simulink model "bh_2dof_NP_CONTROLLED_compare_lagr_sm"  (R2017a)
settings: Solver=ode45  StartTime=0.0  StopTime=70  FixedStep=0.001  RelTol=1e-7  EnableMultiTasking=on
values from neighbouring files (symbols this model uses):
  theta1_0 = 0    [bh_SIMPARAMS_for_2dof_NP_Control_sim.m]
  theta1_dot_0 = 0    [bh_SIMPARAMS_for_2dof_NP_Control_sim.m]
  theta4_0 = 0    [bh_SIMPARAMS_for_2dof_NP_Control_sim.m]
  theta4_dot_0 = 0    [bh_SIMPARAMS_for_2dof_NP_Control_sim.m]
undefined symbols (not defined in the file or in its folder): b1_damp, b4_damp, g, Hz, L1x, L1y, L1z, mass1, mass4, Rturn, sigbuilder_block, X, Y, Z
libraries: simulink_extras x30, sm_lib x13, nesl_utility x9, simulink x8, discretizing x2
(part 1 of 2)
settings Model: Creator=bhorton  LastModifiedBy=bhorton
settings SolverCC: ZeroCrossAlgorithm=Adaptive
settings OptimizationCC: LifeSpan=inf
settings DebuggingCC: SFUnexpectedBacktrackingDiag=warning  SFNoUnconditionalDefaultTransitionDiag=warning  SFExecutionAtInitializationDiag=none
settings GRTTargetCC: TargetLangStandard=C89/C90 (ANSI)
settings ConfigComp: CovMetricSettings=dw  CovHtmlReporting=on  CovSaveCumulativeToWorkspaceVar=on  CovSaveSingleToWorkspaceVar=on  CovExternalEMLEnable=off
settings SimscapeCC: SimscapeLogDataHistory=10000  SelectedTab=Simscape Multibody
settings ExplorerConfigSet: InternalSimMechanicsExplorerSettings="<ExplorerConfiguration><canonicalview>default</canonicalview><AnimationSetting><BasePlaybackSpeed>2</BasePlaybackSpeed><PlaybackSpeedFactor>1.0</PlaybackSpeedFactor></AnimationSetting><TilePanel><TileInfo><Tiles Columns=\"1\" Count=\"1\" Rows=\"1\"><Column Left=\"2\" Weight=\"1\"/><Column Left=\"820\"/><Row Top=\"2\" Weight=\"1\"/><Row Top=\"545\"/><Tile Height=\"1\" Width=\"1\" X=\"0\" Y=\"0\"/></Tiles></TileInfo><SceneInfo><SceneViewer><BGColor><R>0.60000002384185791</R><G>0.60000002384185791</G><B>0.60000002384185791</B></BGColor><Camera><DoPerspective>off</DoPerspective><Position><X>0.3018347345439823</X><Y>0.024415264242792611</Y><Z>0.21433472519445274</Z></Position><Center><X>0.024999999062628675</X><Y>0.30124999972414623</Y><Z>-0.062500010286905439</Z></Center><Up><X>-0.40824829046386751</X><Y>0.40824829046386751</Y><Z>0.81649658092772159</Z></Up><ViewLimDist>1</ViewLimDist><YLim>0.27384785473346712</YLim><XLim>0.4148743716842227</XLim></Camera></SceneViewer></SceneInfo></TilePanel><MechEditorPanel><Cameras/><GfxPanelCameraMap/></MechEditorPanel></ExplorerConfiguration>"

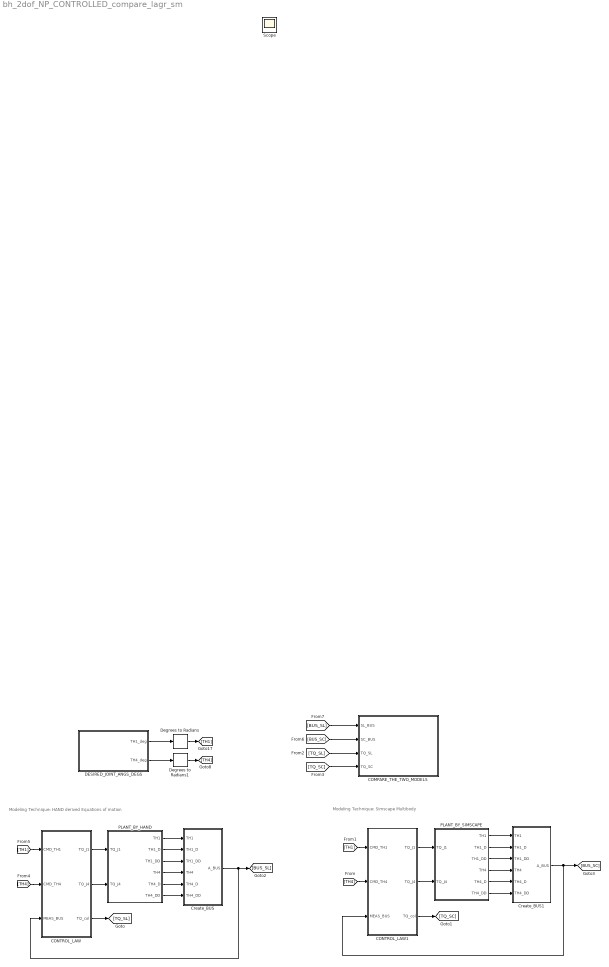
== system bh_2dof_NP_CONTROLLED_compare_lagr_sm ==
  note: Modeling Technique: Simscape Multibody
  note: Modeling Technique: HAND derived Equations of motion
  COMPARE_THE_TWO_MODELS : Subsystem
  CONTROL_LAW : Subsystem
  CONTROL_LAW1 : Subsystem
  Create_BUS : Subsystem
  Create_BUS1 : Subsystem
  DESIRED_JOINT_ANGS_DEGS : Subsystem  Tag=STV Subsys  LoadFcn=sigbuilder_block('load');  StartFcn=sigbuilder_block('start');  StopFcn=sigbuilder_block('stop');  ClipboardFcn=sigbuilder_block('clipboard');  mask(Sigbuilder block){tuvar=[0:10]}
      mask help: Simulink:masks:SigbuilderBlock_MD
      mask init:
      | if ~strcmp(get_param(bdroot(gcbh),'SimulationStatus'),'stopped') tuvar = sigbuilder_block('maskInit'); end
      settings: CopyFcn=sigbuilder_block('copy');  DeleteFcn=sigbuilder_block('delete');  ModelCloseFcn=sigbuilder_block('modelClose');  PreSaveFcn=sigbuilder_block('preSave');  PauseFcn=sigbuilder_block('pause');  ContinueFcn=sigbuilder_block('continue');  NameChangeFcn=sigbuilder_block('namechange');  OpenFcn=sigbuilder_block('open',[6 30 1428 681.75 ]);  CloseFcn=sigbuilder_block('close');
      mask Display: plot(0, 0, 100, 100,[2, 2, 32, 32, 2], [68, 8, 8, 68, 68],[32, 2], [38, 38], [32, 19, 2],[53, 60, 44], [32, 17, 17, 2],[16, 16, 31, 31]);txt = getActiveGroup(gcbh);text(2, 100, txt,'verticalAlignment', 'top');
  Degrees to Radians : simulink_extras/Transformations/Degrees to Radians
  Degrees to Radians1 : simulink_extras/Transformations/Degrees to Radians
  PLANT_BY_HAND : Subsystem
  PLANT_BY_SIMSCAPE : Subsystem
  Scope : Scope
  wires:
  DESIRED_JOINT_ANGS_DEGS/2(TH4_deg) -> Degrees to Radians1/1
  DESIRED_JOINT_ANGS_DEGS/1(TH1_deg) -> Degrees to Radians/1
  Degrees to Radians/1 -> [TH1]
  Degrees to Radians1/1 -> [TH4]
  CONTROL_LAW/1(TQ_J1) -> PLANT_BY_HAND/1("TQ_J1 ")
  Create_BUS/1(A_BUS) -> [BUS_SL], CONTROL_LAW/3(MEAS_BUS)
  PLANT_BY_HAND/4(TH4) -> Create_BUS/4(TH4)
  PLANT_BY_HAND/6(TH4_DD) -> Create_BUS/6(TH4_DD)
  PLANT_BY_HAND/1(TH1) -> Create_BUS/1(TH1)
  PLANT_BY_HAND/2(TH1_D) -> Create_BUS/2(TH1_D)
  PLANT_BY_HAND/3(TH1_DD) -> Create_BUS/3(TH1_DD)
  PLANT_BY_HAND/5(TH4_D) -> Create_BUS/5(TH4_D)
  PLANT_BY_SIMSCAPE/1(TH1) -> Create_BUS1/1(TH1)
  PLANT_BY_SIMSCAPE/2(TH1_D) -> Create_BUS1/2(TH1_D)
  PLANT_BY_SIMSCAPE/3(TH1_DD) -> Create_BUS1/3(TH1_DD)
  PLANT_BY_SIMSCAPE/4(TH4) -> Create_BUS1/4(TH4)
  PLANT_BY_SIMSCAPE/5(TH4_D) -> Create_BUS1/5(TH4_D)
  PLANT_BY_SIMSCAPE/6(TH4_DD) -> Create_BUS1/6(TH4_DD)
  Create_BUS1/1(A_BUS) -> [BUS_SC], CONTROL_LAW1/3(MEAS_BUS)
  CONTROL_LAW1/1(TQ_J1) -> PLANT_BY_SIMSCAPE/1("TQ_J1 ")
  CONTROL_LAW1/2(TQ_J4) -> PLANT_BY_SIMSCAPE/2(TQ_J4)
  [TH4] -> CONTROL_LAW1/2(CMD_TH4)
  [TH1] -> CONTROL_LAW1/1(CMD_TH1)
  CONTROL_LAW/3(TQ_col) -> [TQ_SL]
  CONTROL_LAW1/3(TQ_col) -> [TQ_SC]
  [TQ_SC] -> COMPARE_THE_TWO_MODELS/4(TQ_SC)
  [TQ_SL] -> COMPARE_THE_TWO_MODELS/3(TQ_SL)
  [TH4] -> CONTROL_LAW/2(CMD_TH4)
  [TH1] -> CONTROL_LAW/1(CMD_TH1)
  [BUS_SC] -> COMPARE_THE_TWO_MODELS/2(SC_BUS)
  [BUS_SL] -> COMPARE_THE_TWO_MODELS/1(SL_BUS)
  CONTROL_LAW/2(TQ_J4) -> PLANT_BY_HAND/2(TQ_J4)

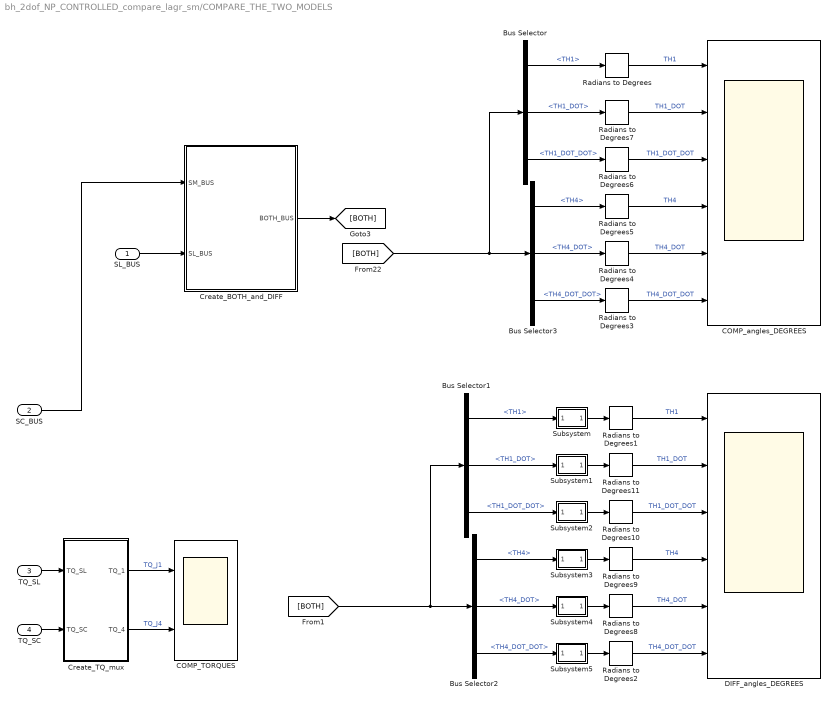
== system bh_2dof_NP_CONTROLLED_compare_lagr_sm/COMPARE_THE_TWO_MODELS ==
  SL_BUS : Inport
  SC_BUS : Inport  Port=2
  TQ_SL : Inport  Port=3
  TQ_SC : Inport  Port=4
  Bus Selector : BusSelector  OutputSignals=TH1,TH1_DOT,TH1_DOT_DOT
  Bus Selector1 : BusSelector  OutputSignals=TH1,TH1_DOT,TH1_DOT_DOT
  Bus Selector2 : BusSelector  OutputSignals=TH4,TH4_DOT,TH4_DOT_DOT
  Bus Selector3 : BusSelector  OutputSignals=TH4,TH4_DOT,TH4_DOT_DOT
  COMP_TORQUES : Scope  NumInputPorts=2
  COMP_angles_DEGREES : Scope  NumInputPorts=6
  Create_BOTH_and_DIFF : Subsystem
  Create_TQ_mux : Subsystem
  DIFF_angles_DEGREES : Scope  NumInputPorts=6
  Radians to Degrees{,1..11} (12 alike) : simulink_extras/Transformations/Radians to Degrees
  Subsystem : Subsystem
  Subsystem1 : Subsystem
  Subsystem2 : Subsystem
  Subsystem3 : Subsystem
  Subsystem4 : Subsystem
  Subsystem5 : Subsystem
  wires:
  SC_BUS/1 -> Create_BOTH_and_DIFF/1(SM_BUS)
  SL_BUS/1 -> Create_BOTH_and_DIFF/2(SL_BUS)
  Create_BOTH_and_DIFF/1(BOTH_BUS) -> [BOTH]
  Bus Selector/1 -> Radians to Degrees/1  "<TH1>"
  Bus Selector/2 -> Radians to Degrees7/1  "<TH1_DOT>"
  Bus Selector/3 -> Radians to Degrees6/1  "<TH1_DOT_DOT>"
  Bus Selector3/1 -> Radians to Degrees5/1  "<TH4>"
  Bus Selector3/2 -> Radians to Degrees4/1  "<TH4_DOT>"
  Bus Selector3/3 -> Radians to Degrees3/1  "<TH4_DOT_DOT>"
  [BOTH] -> Bus Selector/1, Bus Selector3/1
  Radians to Degrees/1 -> COMP_angles_DEGREES/1  "TH1"
  Radians to Degrees7/1 -> COMP_angles_DEGREES/2  "TH1_DOT"
  Radians to Degrees6/1 -> COMP_angles_DEGREES/3  "TH1_DOT_DOT"
  Radians to Degrees5/1 -> COMP_angles_DEGREES/4  "TH4"
  Radians to Degrees4/1 -> COMP_angles_DEGREES/5  "TH4_DOT"
  Radians to Degrees3/1 -> COMP_angles_DEGREES/6  "TH4_DOT_DOT"
  Bus Selector1/1 -> Subsystem/1(In1)  "<TH1>"
  Bus Selector1/2 -> Subsystem1/1(In1)  "<TH1_DOT>"
  Bus Selector1/3 -> Subsystem2/1(In1)  "<TH1_DOT_DOT>"
  Bus Selector2/1 -> Subsystem3/1(In1)  "<TH4>"
  Bus Selector2/2 -> Subsystem4/1(In1)  "<TH4_DOT>"
  Bus Selector2/3 -> Subsystem5/1(In1)  "<TH4_DOT_DOT>"
  [BOTH] -> Bus Selector1/1, Bus Selector2/1
  Radians to Degrees1/1 -> DIFF_angles_DEGREES/1  "TH1"
  Radians to Degrees11/1 -> DIFF_angles_DEGREES/2  "TH1_DOT"
  Radians to Degrees10/1 -> DIFF_angles_DEGREES/3  "TH1_DOT_DOT"
  Radians to Degrees9/1 -> DIFF_angles_DEGREES/4  "TH4"
  Radians to Degrees8/1 -> DIFF_angles_DEGREES/5  "TH4_DOT"
  Radians to Degrees2/1 -> DIFF_angles_DEGREES/6  "TH4_DOT_DOT"
  Subsystem/1(diff) -> Radians to Degrees1/1
  Subsystem5/1(diff) -> Radians to Degrees2/1
  Subsystem4/1(diff) -> Radians to Degrees8/1
  Subsystem3/1(diff) -> Radians to Degrees9/1
  Subsystem2/1(diff) -> Radians to Degrees10/1
  Subsystem1/1(diff) -> Radians to Degrees11/1
  TQ_SC/1 -> Create_TQ_mux/2(TQ_SC)
  TQ_SL/1 -> Create_TQ_mux/1(TQ_SL)
  Create_TQ_mux/1(TQ_1) -> COMP_TORQUES/1  "TQ_J1"
  Create_TQ_mux/2(TQ_4) -> COMP_TORQUES/2  "TQ_J4"

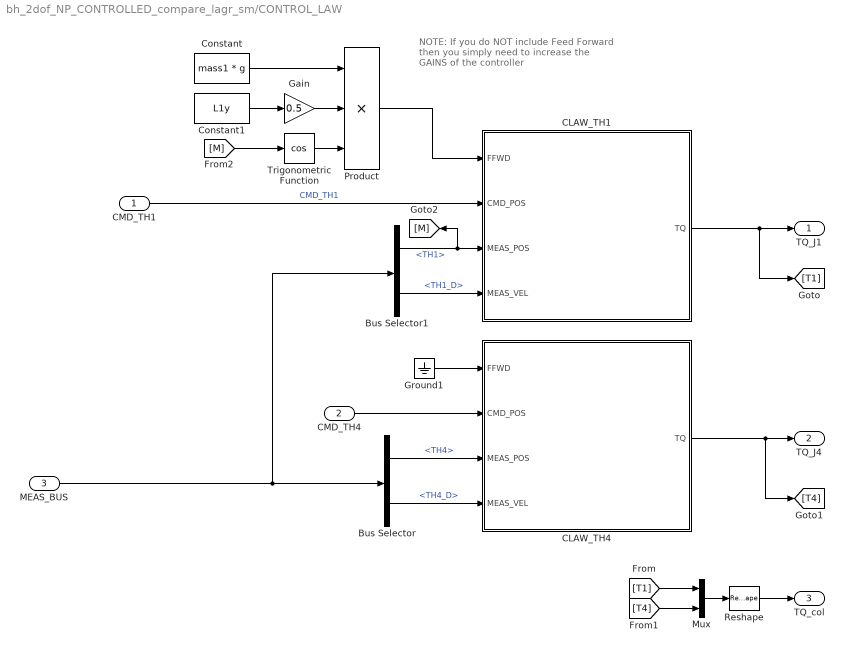
== system bh_2dof_NP_CONTROLLED_compare_lagr_sm/CONTROL_LAW ==
  note: NOTE:
      | If you do NOT include Feed Forward
      | then you simply need to increase the GAINS of the controller
  CMD_TH1 : Inport
  CMD_TH4 : Inport  Port=2
  MEAS_BUS : Inport  Port=3
  Bus Selector : BusSelector  OutputSignals=TH4,TH4_D
  Bus Selector1 : BusSelector  OutputSignals=TH1,TH1_D
  CLAW_TH1 : Subsystem
  CLAW_TH4 : Subsystem
  Constant : Constant  Value=mass1 * g
  Constant1 : Constant  Value=L1y
  Gain : Gain  Gain=0.5
  Ground1 : Ground
  Mux : Mux  Inputs=2
  Product : Product  Inputs=3
  Reshape : Reshape  OutputDimensionality=Column vector (2-D)
  Trigonometric Function : Trigonometry  Operator=cos
  TQ_J1 : Outport
  TQ_J4 : Outport  Port=2
  TQ_col : Outport  Port=3
  wires:
  MEAS_BUS/1 -> Bus Selector1/1, Bus Selector/1
  CMD_TH4/1 -> CLAW_TH4/2(CMD_POS)
  Bus Selector/2 -> CLAW_TH4/4(MEAS_VEL)  "<TH4_D>"
  Bus Selector/1 -> CLAW_TH4/3(MEAS_POS)  "<TH4>"
  Bus Selector1/1 -> [M], CLAW_TH1/3(MEAS_POS)  "<TH1>"
  Bus Selector1/2 -> CLAW_TH1/4(MEAS_VEL)  "<TH1_D>"
  CLAW_TH1/1(TQ) -> [T1], TQ_J1/1
  Ground1/1 -> CLAW_TH4/1(FFWD)
  CLAW_TH4/1(TQ) -> [T4], TQ_J4/1
  CMD_TH1/1 -> CLAW_TH1/2(CMD_POS)  "CMD_TH1"
  Constant/1 -> Product/1
  Constant1/1 -> Gain/1
  Product/1 -> CLAW_TH1/1(FFWD)
  Gain/1 -> Product/2
  Trigonometric Function/1 -> Product/3
  Mux/1 -> Reshape/1
  [T1] -> Mux/1
  [T4] -> Mux/2
  Reshape/1 -> TQ_col/1
  [M] -> Trigonometric Function/1

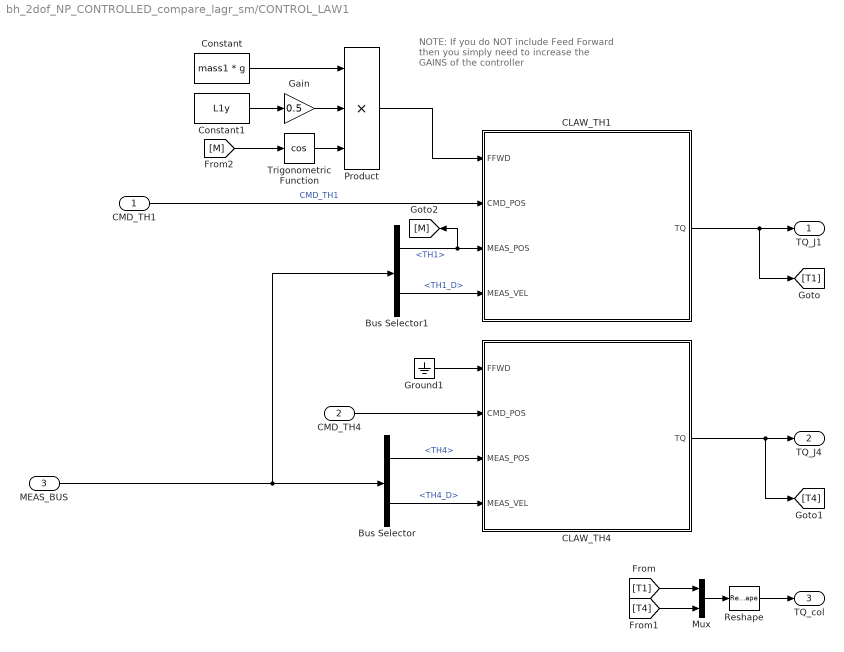
== system bh_2dof_NP_CONTROLLED_compare_lagr_sm/CONTROL_LAW1 ==
  note: NOTE:
      | If you do NOT include Feed Forward
      | then you simply need to increase the GAINS of the controller
  CMD_TH1 : Inport
  CMD_TH4 : Inport  Port=2
  MEAS_BUS : Inport  Port=3
  Bus Selector : BusSelector  OutputSignals=TH4,TH4_D
  Bus Selector1 : BusSelector  OutputSignals=TH1,TH1_D
  CLAW_TH1 : Subsystem
  CLAW_TH4 : Subsystem
  Constant : Constant  Value=mass1 * g
  Constant1 : Constant  Value=L1y
  Gain : Gain  Gain=0.5
  Ground1 : Ground
  Mux : Mux  Inputs=2
  Product : Product  Inputs=3
  Reshape : Reshape  OutputDimensionality=Column vector (2-D)
  Trigonometric Function : Trigonometry  Operator=cos
  TQ_J1 : Outport
  TQ_J4 : Outport  Port=2
  TQ_col : Outport  Port=3
  wires:
  MEAS_BUS/1 -> Bus Selector1/1, Bus Selector/1
  CMD_TH4/1 -> CLAW_TH4/2(CMD_POS)
  Bus Selector/2 -> CLAW_TH4/4(MEAS_VEL)  "<TH4_D>"
  Bus Selector/1 -> CLAW_TH4/3(MEAS_POS)  "<TH4>"
  Bus Selector1/1 -> [M], CLAW_TH1/3(MEAS_POS)  "<TH1>"
  Bus Selector1/2 -> CLAW_TH1/4(MEAS_VEL)  "<TH1_D>"
  CLAW_TH1/1(TQ) -> [T1], TQ_J1/1
  Ground1/1 -> CLAW_TH4/1(FFWD)
  CLAW_TH4/1(TQ) -> [T4], TQ_J4/1
  CMD_TH1/1 -> CLAW_TH1/2(CMD_POS)  "CMD_TH1"
  Constant/1 -> Product/1
  Constant1/1 -> Gain/1
  Product/1 -> CLAW_TH1/1(FFWD)
  Gain/1 -> Product/2
  Trigonometric Function/1 -> Product/3
  Mux/1 -> Reshape/1
  [T1] -> Mux/1
  [T4] -> Mux/2
  Reshape/1 -> TQ_col/1
  [M] -> Trigonometric Function/1

== system bh_2dof_NP_CONTROLLED_compare_lagr_sm/Create_BUS ==
  TH1 : Inport
  TH1_D : Inport  Port=2
  TH1_DD : Inport  Port=3
  TH4 : Inport  Port=4
  TH4_D : Inport  Port=5
  TH4_DD : Inport  Port=6
  Bus Creator : BusCreator  Inputs=6
  A_BUS : Outport
  wires:
  TH1_DD/1 -> Bus Creator/3  "TH1_DD"
  TH1_D/1 -> Bus Creator/2  "TH1_D"
  TH1/1 -> Bus Creator/1  "TH1"
  Bus Creator/1 -> A_BUS/1
  TH4_DD/1 -> Bus Creator/6  "TH4_DD"
  TH4_D/1 -> Bus Creator/5  "TH4_D"
  TH4/1 -> Bus Creator/4  "TH4"

== system bh_2dof_NP_CONTROLLED_compare_lagr_sm/Create_BUS1 ==
  TH1 : Inport
  TH1_D : Inport  Port=2
  TH1_DD : Inport  Port=3
  TH4 : Inport  Port=4
  TH4_D : Inport  Port=5
  TH4_DD : Inport  Port=6
  Bus Creator : BusCreator  Inputs=6
  A_BUS : Outport
  wires:
  TH1_DD/1 -> Bus Creator/3  "TH1_DD"
  TH1_D/1 -> Bus Creator/2  "TH1_D"
  TH1/1 -> Bus Creator/1  "TH1"
  Bus Creator/1 -> A_BUS/1
  TH4_DD/1 -> Bus Creator/6  "TH4_DD"
  TH4_D/1 -> Bus Creator/5  "TH4_D"
  TH4/1 -> Bus Creator/4  "TH4"

== system bh_2dof_NP_CONTROLLED_compare_lagr_sm/DESIRED_JOINT_ANGS_DEGS ==
  Demux : Demux  Tag=STV Demux  Outputs=2
  FromWs : FromWorkspace  Tag=STV FromWs  VariableName=tuvar  SampleTime=0
      SigBuilderData=|
      | common.afterFinalStr = 'Extrapolate'
      | common.sampleTime = 0
      | dataSet(1).timeRange = [0 60]
      | dataSet(1).name = 'SCENARIO_A_JUST_TH1'
      | dataSet(2).timeRange = [0 60]
      | dataSet(2).name = 'SCENARIO_B_JUST_TH4'
      | dataSet(3).timeRange = [0 60]
      | dataSet(3).name = 'SCENARIO_C_TH1_and_TH4'
      | dataSet(4).timeRange = [0 60]
      | dataSet(4).name = 'SCENARIO_D_TH1_and_TH4'
      | dataSet(5).timeRange = [0 70]
      | dataSet(5).name = 'SCENARIO_E'
      | sbobj.Groups(1).Name = 'SCENARIO_A_JUST_TH1'
      | sbobj.Groups(1).Signals(1).Name = 'TH1_deg'
      | sbobj.Groups(1).Signals(1).XData = [0 20 20 60]
      | sbobj.Groups(1).Signals(1).YData = [0 0 45 45]
      | sbobj.Groups(1).Signals(2).Name = 'TH4_deg'
      | sbobj.Groups(1).Signals(2).XData = [0 60]
      | sbobj.Groups(1).Signals(2).YData = [0 0]
      | sbobj.Groups(1).TimeRange = [0 60]
      | sbobj.Groups(2).Name = 'SCENARIO_B_JUST_TH4'
      | sbobj.Groups(2).Signals(1).Name = 'TH1_deg'
      | sbobj.Groups(2).Signals(1).XData = [0 20 60]
      | sbobj.Groups(2).Signals(1).YData = [0 0 0]
      | sbobj.Groups(2).Signals(2).Name = 'TH4_deg'
      | sbobj.Groups(2).Signals(2).XData = [0 20 20 60]
      | sbobj.Groups(2).Signals(2).YData = [0 0 45 45]
      | sbobj.Groups(2).TimeRange = [0 60]
      | sbobj.Groups(3).Name = 'SCENARIO_C_TH1_and_TH4'
      | sbobj.Groups(3).Signals(1).Name = 'TH1_deg'
      | sbobj.Groups(3).Signals(1).XData = [0 10 10 40 60]
      | sbobj.Groups(3).Signals(1).YData = [0 0 45 45 0]
      | sbobj.Groups(3).Signals(2).Name = 'TH4_deg'
      | sbobj.Groups(3).Signals(2).XData = [0 14.95 14.95 30 60]
      | sbobj.Groups(3).Signals(2).YData = [0 0 45 45 0]
      | sbobj.Groups(3).TimeRange = [0 60]
      | sbobj.Groups(4).Name = 'SCENARIO_D_TH1_and_TH4'
      | sbobj.Groups(4).Signals(1).Name = 'TH1_deg'
      | sbobj.Groups(4).Signals(1).XData = [0 10 40 60]
      | sbobj.Groups(4).Signals(1).YData = [0 45 45 0]
      | sbobj.Groups(4).Signals(2).Name = 'TH4_deg'
      | sbobj.Groups(4).Signals(2).XData = [0 10 30 60]
      | sbobj.Groups(4).Signals(2).YData = [0 45 45 0]
      | sbobj.Groups(4).TimeRange = [0 60]
      | sbobj.Groups(5).Name = 'SCENARIO_E'
      | sbobj.Groups(5).Signals(1).Name = 'TH1_deg'
      | sbobj.Groups(5).Signals(1).XData = [0 35.15 45.4 60 70]
      | sbobj.Groups(5).Signals(1).YData = [0 0 45 -45 0]
      | sbobj.Groups(5).Signals(2).Name = 'TH4_deg'
      | sbobj.Groups(5).Signals(2).XData = [0 10 25 30 70]
      | sbobj.Groups(5).Signals(2).YData = [0 -90 90 0 0]
      | sbobj.Groups(5).TimeRange = [0 70]
  TH1_deg : Outport  Tag=STV Outport
  TH4_deg : Outport  Tag=STV Outport  Port=2
  wires:
  FromWs/1 -> Demux/1
  Demux/1 -> TH1_deg/1
  Demux/2 -> TH4_deg/1

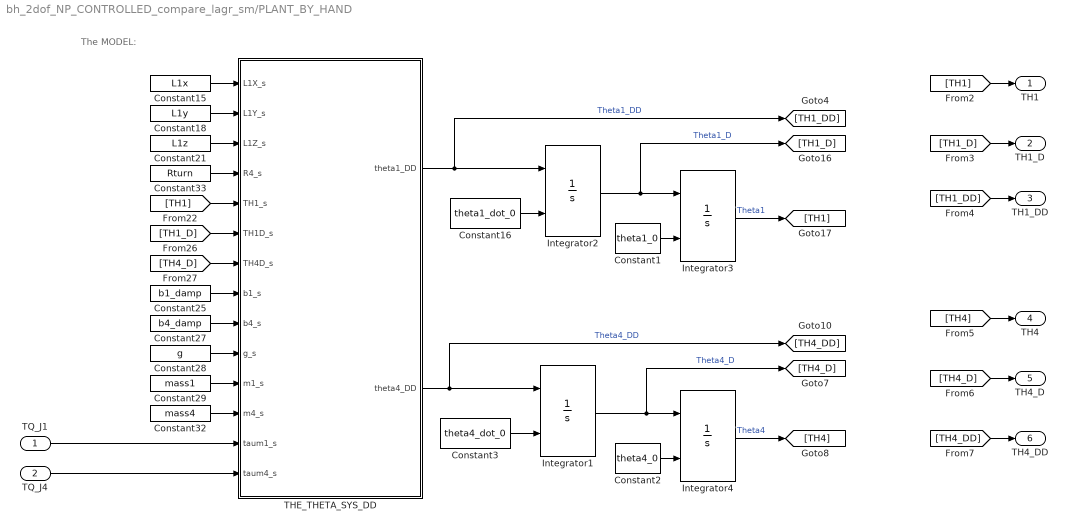
== system bh_2dof_NP_CONTROLLED_compare_lagr_sm/PLANT_BY_HAND ==
  note: The MODEL:
  "TQ_J1 " : Inport
  TQ_J4 : Inport  Port=2
  Constant1 : Constant  Value=theta1_0
  Constant15 : Constant  Value=L1x
  Constant16 : Constant  Value=theta1_dot_0
  Constant18 : Constant  Value=L1y
  Constant2 : Constant  Value=theta4_0
  Constant21 : Constant  Value=L1z
  Constant25 : Constant  Value=b1_damp
  Constant27 : Constant  Value=b4_damp
  Constant28 : Constant  Value=g
  Constant29 : Constant  Value=mass1
  Constant3 : Constant  Value=theta4_dot_0
  Constant32 : Constant  Value=mass4
  Constant33 : Constant  Value=Rturn
  Integrator{1..4} (4 alike) : Integrator  InitialConditionSource=external
  THE_THETA_SYS_DD : MATLAB Function  TreatAsAtomicUnit=on
  TH1 : Outport
  TH1_D : Outport  Port=2
  TH1_DD : Outport  Port=3
  TH4 : Outport  Port=4
  TH4_D : Outport  Port=5
  TH4_DD : Outport  Port=6
  wires:
  [TH4_D] -> TH4_D/1
  Constant16/1 -> Integrator2/2
  Integrator2/1 -> [TH1_D], Integrator3/1  "Theta1_D"
  TQ_J4/1 -> THE_THETA_SYS_DD/14(taum4_s)
  Integrator4/1 -> [TH4]  "Theta4"
  [TH4_D] -> THE_THETA_SYS_DD/7(TH4D_s)
  [TH1] -> THE_THETA_SYS_DD/5(TH1_s)
  [TH1_DD] -> TH1_DD/1
  Constant29/1 -> THE_THETA_SYS_DD/11(m1_s)
  Constant33/1 -> THE_THETA_SYS_DD/4(R4_s)
  THE_THETA_SYS_DD/1(theta1_DD) -> [TH1_DD], Integrator2/1  "Theta1_DD"
  Integrator3/1 -> [TH1]  "Theta1"
  Constant18/1 -> THE_THETA_SYS_DD/2(L1Y_s)
  THE_THETA_SYS_DD/2(theta4_DD) -> Integrator1/1, [TH4_DD]  "Theta4_DD"
  Constant2/1 -> Integrator4/2
  "TQ_J1 "/1 -> THE_THETA_SYS_DD/13(taum1_s)
  [TH1] -> TH1/1
  Constant1/1 -> Integrator3/2
  Constant27/1 -> THE_THETA_SYS_DD/9(b4_s)
  [TH1_D] -> TH1_D/1
  Constant32/1 -> THE_THETA_SYS_DD/12(m4_s)
  [TH4_DD] -> TH4_DD/1
  Constant3/1 -> Integrator1/2
  Constant25/1 -> THE_THETA_SYS_DD/8(b1_s)
  [TH4] -> TH4/1
  Constant15/1 -> THE_THETA_SYS_DD/1(L1X_s)
  Constant21/1 -> THE_THETA_SYS_DD/3(L1Z_s)
  [TH1_D] -> THE_THETA_SYS_DD/6(TH1D_s)
  Integrator1/1 -> [TH4_D], Integrator4/1  "Theta4_D"
  Constant28/1 -> THE_THETA_SYS_DD/10(g_s)

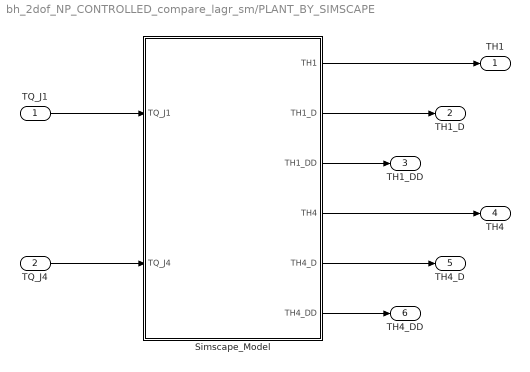
== system bh_2dof_NP_CONTROLLED_compare_lagr_sm/PLANT_BY_SIMSCAPE ==
  "TQ_J1 " : Inport
  TQ_J4 : Inport  Port=2
  Simscape_Model : Subsystem  VariantControl=Variant1
  TH1 : Outport
  TH1_D : Outport  Port=2
  TH1_DD : Outport  Port=3
  TH4 : Outport  Port=4
  TH4_D : Outport  Port=5
  TH4_DD : Outport  Port=6
  wires:
  TQ_J4/1 -> Simscape_Model/2(TQ_J4)
  "TQ_J1 "/1 -> Simscape_Model/1("TQ_J1 ")
  Simscape_Model/1(TH1) -> TH1/1
  Simscape_Model/2(TH1_D) -> TH1_D/1
  Simscape_Model/3(TH1_DD) -> TH1_DD/1
  Simscape_Model/6(TH4_DD) -> TH4_DD/1
  Simscape_Model/5(TH4_D) -> TH4_D/1
  Simscape_Model/4(TH4) -> TH4/1

== system bh_2dof_NP_CONTROLLED_compare_lagr_sm/COMPARE_THE_TWO_MODELS/Create_BOTH_and_DIFF ==
  SM_BUS : Inport
  SL_BUS : Inport  Port=2
  BOTH : Subsystem
  BOTH_BUS : Outport
  wires:
  SL_BUS/1 -> [SL_BUS]
  SM_BUS/1 -> [SM_BUS]
  [SM_BUS] -> BOTH/1(SM_BUS)
  [SL_BUS] -> BOTH/2(SL_BUS)
  BOTH/1(BOTH_BUS) -> BOTH_BUS/1

== system bh_2dof_NP_CONTROLLED_compare_lagr_sm/COMPARE_THE_TWO_MODELS/Create_TQ_mux ==
  TQ_SL : Inport
  TQ_SC : Inport  Port=2
  Mux : Mux  Inputs=2
  Selector : Selector  InputPortWidth=4  IndexOptions=Index vector (dialog)  Indices=[1 3]  OutputSizes=1
  Selector1 : Selector  InputPortWidth=4  IndexOptions=Index vector (dialog)  Indices=[2 4]  OutputSizes=1
  TQ_1 : Outport
  TQ_4 : Outport  Port=2
  wires:
  TQ_SL/1 -> Mux/1
  TQ_SC/1 -> Mux/2
  Mux/1 -> Selector1/1, Selector/1
  Selector/1 -> TQ_1/1
  Selector1/1 -> TQ_4/1

== system bh_2dof_NP_CONTROLLED_compare_lagr_sm/COMPARE_THE_TWO_MODELS/Subsystem ==
  In1 : Inport
  Demux : Demux  Outputs=2
  Sum : Sum  Inputs=|+-
  diff : Outport
  wires:
  In1/1 -> Demux/1
  Demux/1 -> Sum/1
  Demux/2 -> Sum/2
  Sum/1 -> diff/1

== system bh_2dof_NP_CONTROLLED_compare_lagr_sm/COMPARE_THE_TWO_MODELS/Subsystem1 ==
  In1 : Inport
  Demux : Demux  Outputs=2
  Sum : Sum  Inputs=|+-
  diff : Outport
  wires:
  In1/1 -> Demux/1
  Demux/1 -> Sum/1
  Demux/2 -> Sum/2
  Sum/1 -> diff/1

== system bh_2dof_NP_CONTROLLED_compare_lagr_sm/COMPARE_THE_TWO_MODELS/Subsystem2 ==
  In1 : Inport
  Demux : Demux  Outputs=2
  Sum : Sum  Inputs=|+-
  diff : Outport
  wires:
  In1/1 -> Demux/1
  Demux/1 -> Sum/1
  Demux/2 -> Sum/2
  Sum/1 -> diff/1

== system bh_2dof_NP_CONTROLLED_compare_lagr_sm/COMPARE_THE_TWO_MODELS/Subsystem3 ==
  In1 : Inport
  Demux : Demux  Outputs=2
  Sum : Sum  Inputs=|+-
  diff : Outport
  wires:
  In1/1 -> Demux/1
  Demux/1 -> Sum/1
  Demux/2 -> Sum/2
  Sum/1 -> diff/1

== system bh_2dof_NP_CONTROLLED_compare_lagr_sm/COMPARE_THE_TWO_MODELS/Subsystem4 ==
  In1 : Inport
  Demux : Demux  Outputs=2
  Sum : Sum  Inputs=|+-
  diff : Outport
  wires:
  In1/1 -> Demux/1
  Demux/1 -> Sum/1
  Demux/2 -> Sum/2
  Sum/1 -> diff/1

== system bh_2dof_NP_CONTROLLED_compare_lagr_sm/COMPARE_THE_TWO_MODELS/Subsystem5 ==
  In1 : Inport
  Demux : Demux  Outputs=2
  Sum : Sum  Inputs=|+-
  diff : Outport
  wires:
  In1/1 -> Demux/1
  Demux/1 -> Sum/1
  Demux/2 -> Sum/2
  Sum/1 -> diff/1

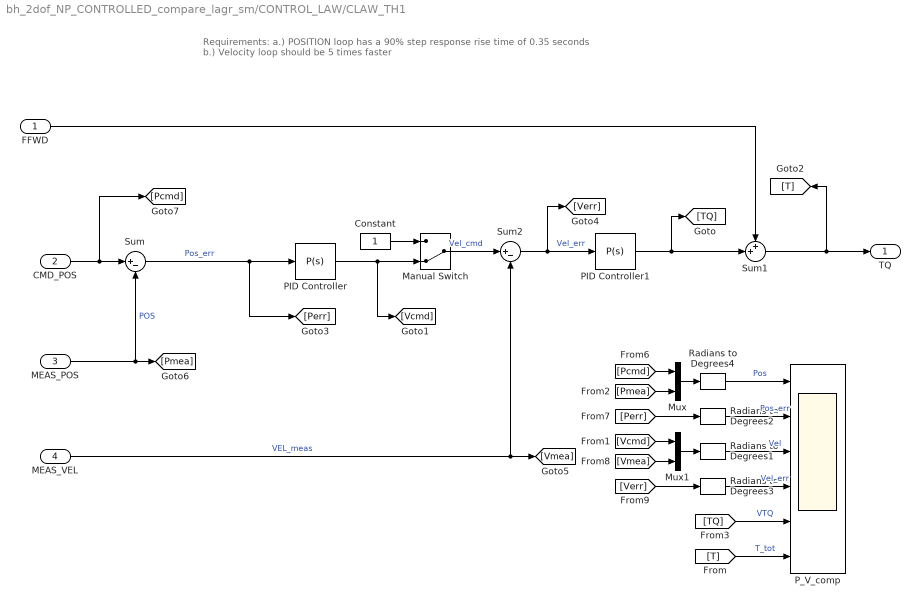
== system bh_2dof_NP_CONTROLLED_compare_lagr_sm/CONTROL_LAW/CLAW_TH1 ==
  note: Requirements:
      | a.) POSITION loop has a 90% step response
      | rise time of 0.35 seconds
      |
      | b.) Velocity loop should be 5 times faster
  FFWD : Inport
  CMD_POS : Inport  Port=2
  MEAS_POS : Inport  Port=3
  MEAS_VEL : Inport  Port=4
  Constant : Constant
  Manual Switch : ManualSwitch  CurrentSetting=0
  Mux : Mux  Inputs=2
  Mux1 : Mux  Inputs=2
  PID Controller : simulink/Continuous/PID Controller  Controller=P  TimeDomain=Continuous-time  SampleTime=-1  IntegratorMethod=Forward Euler  FilterMethod=Forward Euler  Form=Parallel  UseFilter=on  ControllerParametersSource=internal  P=5.58549433794614  I=0  D=0  N=100  InitialConditionSource=internal  InitialConditionForIntegrator=0  InitialConditionForFilter=0  ExternalReset=none  LimitOutput=off  UpperSaturationLimit=inf  LowerSaturationLimit=-inf  LinearizeAsGain=on  AntiWindupMode=none  Kb=1  TrackingMode=off  Kt=1  PParamMin=[]  PParamMax=[]  IParamMin=[]  IParamMax=[]  DParamMin=[]  DParamMax=[]  NParamMin=[]  NParamMax=[]  KbParamMin=[]  KbParamMax=[]  KtParamMin=[]  KtParamMax=[]  POutMin=[]  POutMax=[]  IOutMin=[]  IOutMax=[]  DOutMin=[]  DOutMax=[]  NOutMin=[]  NOutMax=[]  KbOutMin=[]  KbOutMax=[]  KtOutMin=[]  KtOutMax=[]  IntegratorOutMin=[]  IntegratorOutMax=[]  FilterOutMin=[]  FilterOutMax=[]  SumOutMin=[]  SumOutMax=[]  SumI1OutMin=[]  SumI1OutMax=[]  SumI2OutMin=[]  SumI2OutMax=[]  SumI3OutMin=[]  SumI3OutMax=[]  SumDOutMin=[]  SumDOutMax=[]  SaturationOutMin=[]  SaturationOutMax=[]  IntegratorContinuousStateAttributes=''  IntegratorStateMustResolveToSignalObject=off  IntegratorRTWStateStorageClass=Auto  FilterContinuousStateAttributes=''  FilterStateMustResolveToSignalObject=off  FilterRTWStateStorageClass=Auto  DifferentiatorICPrevScaledInput=0  DifferentiatorOutMin=[]  DifferentiatorOutMax=[]  InitialConditionSetting=State (most efficient)
  PID Controller1 : simulink/Continuous/PID Controller  Controller=P  TimeDomain=Continuous-time  SampleTime=-1  IntegratorMethod=Forward Euler  FilterMethod=Forward Euler  Form=Parallel  UseFilter=on  ControllerParametersSource=internal  P=1  I=1  D=0  N=100  InitialConditionSource=internal  InitialConditionForIntegrator=0  InitialConditionForFilter=0  ExternalReset=none  LimitOutput=off  UpperSaturationLimit=inf  LowerSaturationLimit=-inf  LinearizeAsGain=on  AntiWindupMode=none  Kb=1  TrackingMode=off  Kt=1  PParamMin=[]  PParamMax=[]  IParamMin=[]  IParamMax=[]  DParamMin=[]  DParamMax=[]  NParamMin=[]  NParamMax=[]  KbParamMin=[]  KbParamMax=[]  KtParamMin=[]  KtParamMax=[]  POutMin=[]  POutMax=[]  IOutMin=[]  IOutMax=[]  DOutMin=[]  DOutMax=[]  NOutMin=[]  NOutMax=[]  KbOutMin=[]  KbOutMax=[]  KtOutMin=[]  KtOutMax=[]  IntegratorOutMin=[]  IntegratorOutMax=[]  FilterOutMin=[]  FilterOutMax=[]  SumOutMin=[]  SumOutMax=[]  SumI1OutMin=[]  SumI1OutMax=[]  SumI2OutMin=[]  SumI2OutMax=[]  SumI3OutMin=[]  SumI3OutMax=[]  SumDOutMin=[]  SumDOutMax=[]  SaturationOutMin=[]  SaturationOutMax=[]  IntegratorContinuousStateAttributes=''  IntegratorStateMustResolveToSignalObject=off  IntegratorRTWStateStorageClass=Auto  FilterContinuousStateAttributes=''  FilterStateMustResolveToSignalObject=off  FilterRTWStateStorageClass=Auto  DifferentiatorICPrevScaledInput=0  DifferentiatorOutMin=[]  DifferentiatorOutMax=[]  InitialConditionSetting=State (most efficient)
  P_V_comp : Scope  NumInputPorts=6
  Radians to Degrees{1..4} (4 alike) : simulink_extras/Transformations/Radians to Degrees
  Sum : Sum  Inputs=|+-
  Sum1 : Sum  Inputs=++|
  Sum2 : Sum  Inputs=|+-
  TQ : Outport
  wires:
  FFWD/1 -> Sum1/1
  CMD_POS/1 -> [Pcmd], Sum/1
  MEAS_VEL/1 -> [Vmea], Sum2/2  "VEL_meas"
  MEAS_POS/1 -> [Pmea], Sum/2  "POS"
  Sum2/1 -> PID Controller1/1, [Verr]  "Vel_err"
  Manual Switch/1 -> Sum2/1  "Vel_cmd"
  Constant/1 -> Manual Switch/1
  Sum/1 -> PID Controller/1, [Perr]  "Pos_err"
  PID Controller/1 -> Manual Switch/2, [Vcmd]
  Sum1/1 -> TQ/1, [T]
  Mux/1 -> Radians to Degrees4/1
  [Pcmd] -> Mux/1
  [Pmea] -> Mux/2
  Mux1/1 -> Radians to Degrees1/1
  [Vcmd] -> Mux1/1
  [Vmea] -> Mux1/2
  [Verr] -> Radians to Degrees3/1
  [Perr] -> Radians to Degrees2/1
  Radians to Degrees3/1 -> P_V_comp/4  "Vel_err"
  Radians to Degrees2/1 -> P_V_comp/2  "Pos_err"
  Radians to Degrees1/1 -> P_V_comp/3  "Vel"
  Radians to Degrees4/1 -> P_V_comp/1  "Pos"
  [TQ] -> P_V_comp/5  "VTQ"
  [T] -> P_V_comp/6  "T_tot"
  PID Controller1/1 -> Sum1/2, [TQ]

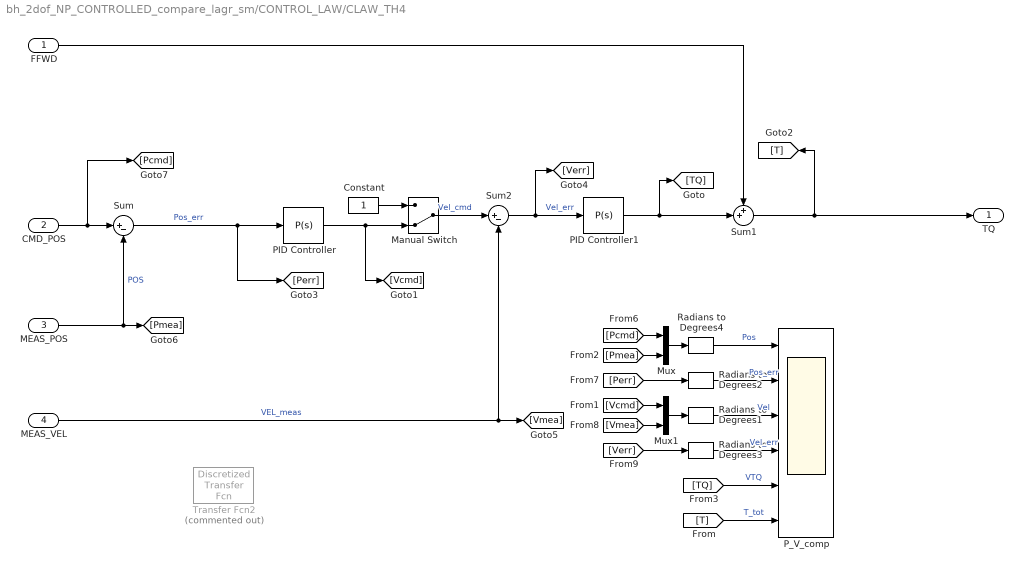
== system bh_2dof_NP_CONTROLLED_compare_lagr_sm/CONTROL_LAW/CLAW_TH4 ==
  FFWD : Inport
  CMD_POS : Inport  Port=2
  MEAS_POS : Inport  Port=3
  MEAS_VEL : Inport  Port=4
  Constant : Constant
  Manual Switch : ManualSwitch  CurrentSetting=0
  Mux : Mux  Inputs=2
  Mux1 : Mux  Inputs=2
  PID Controller : simulink/Continuous/PID Controller  Controller=P  TimeDomain=Continuous-time  SampleTime=-1  IntegratorMethod=Forward Euler  FilterMethod=Forward Euler  Form=Parallel  UseFilter=on  ControllerParametersSource=internal  P=5.58549433794614  I=1  D=0  N=100  InitialConditionSource=internal  InitialConditionForIntegrator=0  InitialConditionForFilter=0  ExternalReset=none  LimitOutput=off  UpperSaturationLimit=inf  LowerSaturationLimit=-inf  LinearizeAsGain=on  AntiWindupMode=none  Kb=1  TrackingMode=off  Kt=1  PParamMin=[]  PParamMax=[]  IParamMin=[]  IParamMax=[]  DParamMin=[]  DParamMax=[]  NParamMin=[]  NParamMax=[]  KbParamMin=[]  KbParamMax=[]  KtParamMin=[]  KtParamMax=[]  POutMin=[]  POutMax=[]  IOutMin=[]  IOutMax=[]  DOutMin=[]  DOutMax=[]  NOutMin=[]  NOutMax=[]  KbOutMin=[]  KbOutMax=[]  KtOutMin=[]  KtOutMax=[]  IntegratorOutMin=[]  IntegratorOutMax=[]  FilterOutMin=[]  FilterOutMax=[]  SumOutMin=[]  SumOutMax=[]  SumI1OutMin=[]  SumI1OutMax=[]  SumI2OutMin=[]  SumI2OutMax=[]  SumI3OutMin=[]  SumI3OutMax=[]  SumDOutMin=[]  SumDOutMax=[]  SaturationOutMin=[]  SaturationOutMax=[]  IntegratorContinuousStateAttributes=''  IntegratorStateMustResolveToSignalObject=off  IntegratorRTWStateStorageClass=Auto  FilterContinuousStateAttributes=''  FilterStateMustResolveToSignalObject=off  FilterRTWStateStorageClass=Auto  DifferentiatorICPrevScaledInput=0  DifferentiatorOutMin=[]  DifferentiatorOutMax=[]  InitialConditionSetting=State (most efficient)
  PID Controller1 : simulink/Continuous/PID Controller  Controller=P  TimeDomain=Continuous-time  SampleTime=-1  IntegratorMethod=Forward Euler  FilterMethod=Forward Euler  Form=Parallel  UseFilter=on  ControllerParametersSource=internal  P=1  I=1  D=0  N=100  InitialConditionSource=internal  InitialConditionForIntegrator=0  InitialConditionForFilter=0  ExternalReset=none  LimitOutput=off  UpperSaturationLimit=inf  LowerSaturationLimit=-inf  LinearizeAsGain=on  AntiWindupMode=none  Kb=1  TrackingMode=off  Kt=1  PParamMin=[]  PParamMax=[]  IParamMin=[]  IParamMax=[]  DParamMin=[]  DParamMax=[]  NParamMin=[]  NParamMax=[]  KbParamMin=[]  KbParamMax=[]  KtParamMin=[]  KtParamMax=[]  POutMin=[]  POutMax=[]  IOutMin=[]  IOutMax=[]  DOutMin=[]  DOutMax=[]  NOutMin=[]  NOutMax=[]  KbOutMin=[]  KbOutMax=[]  KtOutMin=[]  KtOutMax=[]  IntegratorOutMin=[]  IntegratorOutMax=[]  FilterOutMin=[]  FilterOutMax=[]  SumOutMin=[]  SumOutMax=[]  SumI1OutMin=[]  SumI1OutMax=[]  SumI2OutMin=[]  SumI2OutMax=[]  SumI3OutMin=[]  SumI3OutMax=[]  SumDOutMin=[]  SumDOutMax=[]  SaturationOutMin=[]  SaturationOutMax=[]  IntegratorContinuousStateAttributes=''  IntegratorStateMustResolveToSignalObject=off  IntegratorRTWStateStorageClass=Auto  FilterContinuousStateAttributes=''  FilterStateMustResolveToSignalObject=off  FilterRTWStateStorageClass=Auto  DifferentiatorICPrevScaledInput=0  DifferentiatorOutMin=[]  DifferentiatorOutMax=[]  InitialConditionSetting=State (most efficient)
  P_V_comp : Scope  NumInputPorts=6
  Radians to Degrees{1..4} (4 alike) : simulink_extras/Transformations/Radians to Degrees
  Sum : Sum  Inputs=|+-
  Sum1 : Sum  Inputs=++|
  Sum2 : Sum  Inputs=|+-
  Transfer Fcn2 : discretizing/Discretized Transfer Fcn  Commented=on  Numerator=[100]  Denominator=[1 100]  AbsTol=auto  SampleTime=0.001  method=tustin  Wc=1
  TQ : Outport
  wires:
  FFWD/1 -> Sum1/1
  CMD_POS/1 -> [Pcmd], Sum/1
  MEAS_VEL/1 -> [Vmea], Sum2/2  "VEL_meas"
  MEAS_POS/1 -> [Pmea], Sum/2  "POS"
  Sum2/1 -> PID Controller1/1, [Verr]  "Vel_err"
  Manual Switch/1 -> Sum2/1  "Vel_cmd"
  Constant/1 -> Manual Switch/1
  Sum/1 -> PID Controller/1, [Perr]  "Pos_err"
  PID Controller/1 -> Manual Switch/2, [Vcmd]
  Sum1/1 -> TQ/1, [T]
  Mux/1 -> Radians to Degrees4/1
  [Pcmd] -> Mux/1
  [Pmea] -> Mux/2
  Mux1/1 -> Radians to Degrees1/1
  [Vcmd] -> Mux1/1
  [Vmea] -> Mux1/2
  [Verr] -> Radians to Degrees3/1
  [Perr] -> Radians to Degrees2/1
  Radians to Degrees3/1 -> P_V_comp/4  "Vel_err"
  Radians to Degrees2/1 -> P_V_comp/2  "Pos_err"
  Radians to Degrees1/1 -> P_V_comp/3  "Vel"
  Radians to Degrees4/1 -> P_V_comp/1  "Pos"
  [TQ] -> P_V_comp/5  "VTQ"
  [T] -> P_V_comp/6  "T_tot"
  PID Controller1/1 -> Sum1/2, [TQ]

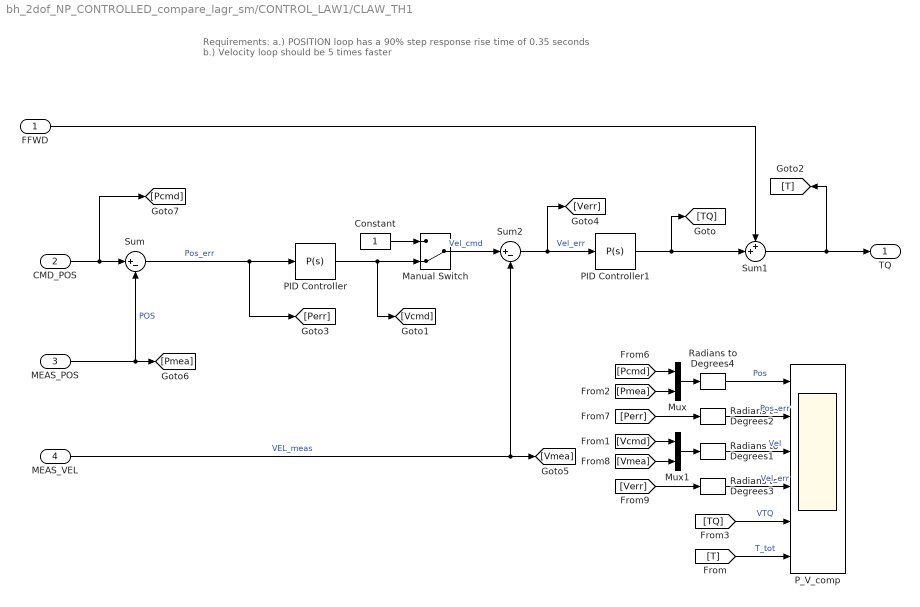
== system bh_2dof_NP_CONTROLLED_compare_lagr_sm/CONTROL_LAW1/CLAW_TH1 ==
  note: Requirements:
      | a.) POSITION loop has a 90% step response
      | rise time of 0.35 seconds
      |
      | b.) Velocity loop should be 5 times faster
  FFWD : Inport
  CMD_POS : Inport  Port=2
  MEAS_POS : Inport  Port=3
  MEAS_VEL : Inport  Port=4
  Constant : Constant
  Manual Switch : ManualSwitch  CurrentSetting=0
  Mux : Mux  Inputs=2
  Mux1 : Mux  Inputs=2
  PID Controller : simulink/Continuous/PID Controller  Controller=P  TimeDomain=Continuous-time  SampleTime=-1  IntegratorMethod=Forward Euler  FilterMethod=Forward Euler  Form=Parallel  UseFilter=on  ControllerParametersSource=internal  P=5.58549433794614  I=0  D=0  N=100  InitialConditionSource=internal  InitialConditionForIntegrator=0  InitialConditionForFilter=0  ExternalReset=none  LimitOutput=off  UpperSaturationLimit=inf  LowerSaturationLimit=-inf  LinearizeAsGain=on  AntiWindupMode=none  Kb=1  TrackingMode=off  Kt=1  PParamMin=[]  PParamMax=[]  IParamMin=[]  IParamMax=[]  DParamMin=[]  DParamMax=[]  NParamMin=[]  NParamMax=[]  KbParamMin=[]  KbParamMax=[]  KtParamMin=[]  KtParamMax=[]  POutMin=[]  POutMax=[]  IOutMin=[]  IOutMax=[]  DOutMin=[]  DOutMax=[]  NOutMin=[]  NOutMax=[]  KbOutMin=[]  KbOutMax=[]  KtOutMin=[]  KtOutMax=[]  IntegratorOutMin=[]  IntegratorOutMax=[]  FilterOutMin=[]  FilterOutMax=[]  SumOutMin=[]  SumOutMax=[]  SumI1OutMin=[]  SumI1OutMax=[]  SumI2OutMin=[]  SumI2OutMax=[]  SumI3OutMin=[]  SumI3OutMax=[]  SumDOutMin=[]  SumDOutMax=[]  SaturationOutMin=[]  SaturationOutMax=[]  IntegratorContinuousStateAttributes=''  IntegratorStateMustResolveToSignalObject=off  IntegratorRTWStateStorageClass=Auto  FilterContinuousStateAttributes=''  FilterStateMustResolveToSignalObject=off  FilterRTWStateStorageClass=Auto  DifferentiatorICPrevScaledInput=0  DifferentiatorOutMin=[]  DifferentiatorOutMax=[]  InitialConditionSetting=State (most efficient)
  PID Controller1 : simulink/Continuous/PID Controller  Controller=P  TimeDomain=Continuous-time  SampleTime=-1  IntegratorMethod=Forward Euler  FilterMethod=Forward Euler  Form=Parallel  UseFilter=on  ControllerParametersSource=internal  P=1  I=1  D=0  N=100  InitialConditionSource=internal  InitialConditionForIntegrator=0  InitialConditionForFilter=0  ExternalReset=none  LimitOutput=off  UpperSaturationLimit=inf  LowerSaturationLimit=-inf  LinearizeAsGain=on  AntiWindupMode=none  Kb=1  TrackingMode=off  Kt=1  PParamMin=[]  PParamMax=[]  IParamMin=[]  IParamMax=[]  DParamMin=[]  DParamMax=[]  NParamMin=[]  NParamMax=[]  KbParamMin=[]  KbParamMax=[]  KtParamMin=[]  KtParamMax=[]  POutMin=[]  POutMax=[]  IOutMin=[]  IOutMax=[]  DOutMin=[]  DOutMax=[]  NOutMin=[]  NOutMax=[]  KbOutMin=[]  KbOutMax=[]  KtOutMin=[]  KtOutMax=[]  IntegratorOutMin=[]  IntegratorOutMax=[]  FilterOutMin=[]  FilterOutMax=[]  SumOutMin=[]  SumOutMax=[]  SumI1OutMin=[]  SumI1OutMax=[]  SumI2OutMin=[]  SumI2OutMax=[]  SumI3OutMin=[]  SumI3OutMax=[]  SumDOutMin=[]  SumDOutMax=[]  SaturationOutMin=[]  SaturationOutMax=[]  IntegratorContinuousStateAttributes=''  IntegratorStateMustResolveToSignalObject=off  IntegratorRTWStateStorageClass=Auto  FilterContinuousStateAttributes=''  FilterStateMustResolveToSignalObject=off  FilterRTWStateStorageClass=Auto  DifferentiatorICPrevScaledInput=0  DifferentiatorOutMin=[]  DifferentiatorOutMax=[]  InitialConditionSetting=State (most efficient)
  P_V_comp : Scope  NumInputPorts=6
  Radians to Degrees{1..4} (4 alike) : simulink_extras/Transformations/Radians to Degrees
  Sum : Sum  Inputs=|+-
  Sum1 : Sum  Inputs=++|
  Sum2 : Sum  Inputs=|+-
  TQ : Outport
  wires:
  FFWD/1 -> Sum1/1
  CMD_POS/1 -> [Pcmd], Sum/1
  MEAS_VEL/1 -> [Vmea], Sum2/2  "VEL_meas"
  MEAS_POS/1 -> [Pmea], Sum/2  "POS"
  Sum2/1 -> PID Controller1/1, [Verr]  "Vel_err"
  Manual Switch/1 -> Sum2/1  "Vel_cmd"
  Constant/1 -> Manual Switch/1
  Sum/1 -> PID Controller/1, [Perr]  "Pos_err"
  PID Controller/1 -> Manual Switch/2, [Vcmd]
  Sum1/1 -> TQ/1, [T]
  Mux/1 -> Radians to Degrees4/1
  [Pcmd] -> Mux/1
  [Pmea] -> Mux/2
  Mux1/1 -> Radians to Degrees1/1
  [Vcmd] -> Mux1/1
  [Vmea] -> Mux1/2
  [Verr] -> Radians to Degrees3/1
  [Perr] -> Radians to Degrees2/1
  Radians to Degrees3/1 -> P_V_comp/4  "Vel_err"
  Radians to Degrees2/1 -> P_V_comp/2  "Pos_err"
  Radians to Degrees1/1 -> P_V_comp/3  "Vel"
  Radians to Degrees4/1 -> P_V_comp/1  "Pos"
  [TQ] -> P_V_comp/5  "VTQ"
  [T] -> P_V_comp/6  "T_tot"
  PID Controller1/1 -> Sum1/2, [TQ]

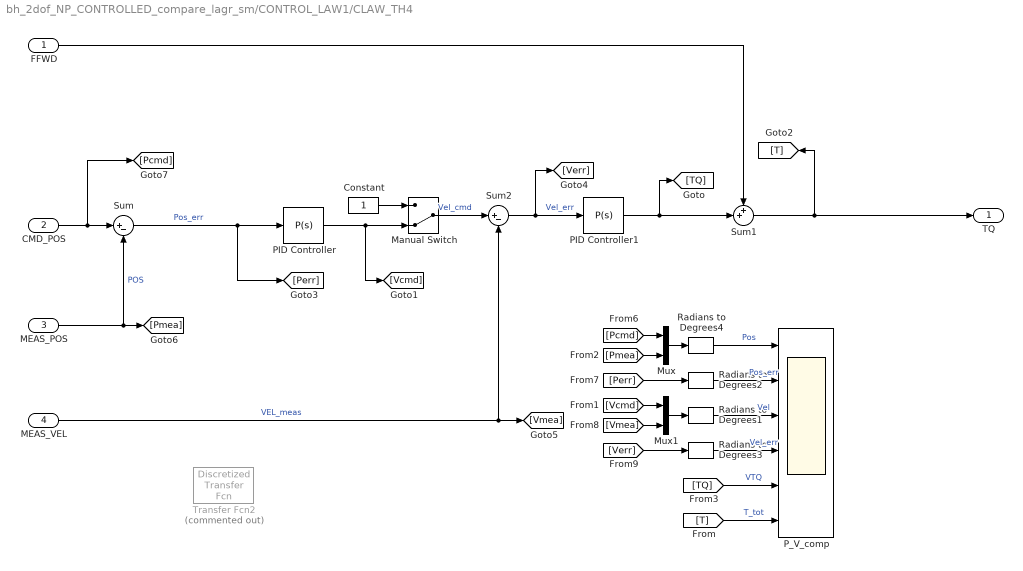
== system bh_2dof_NP_CONTROLLED_compare_lagr_sm/CONTROL_LAW1/CLAW_TH4 ==
  FFWD : Inport
  CMD_POS : Inport  Port=2
  MEAS_POS : Inport  Port=3
  MEAS_VEL : Inport  Port=4
  Constant : Constant
  Manual Switch : ManualSwitch  CurrentSetting=0
  Mux : Mux  Inputs=2
  Mux1 : Mux  Inputs=2
  PID Controller : simulink/Continuous/PID Controller  Controller=P  TimeDomain=Continuous-time  SampleTime=-1  IntegratorMethod=Forward Euler  FilterMethod=Forward Euler  Form=Parallel  UseFilter=on  ControllerParametersSource=internal  P=5.58549433794614  I=1  D=0  N=100  InitialConditionSource=internal  InitialConditionForIntegrator=0  InitialConditionForFilter=0  ExternalReset=none  LimitOutput=off  UpperSaturationLimit=inf  LowerSaturationLimit=-inf  LinearizeAsGain=on  AntiWindupMode=none  Kb=1  TrackingMode=off  Kt=1  PParamMin=[]  PParamMax=[]  IParamMin=[]  IParamMax=[]  DParamMin=[]  DParamMax=[]  NParamMin=[]  NParamMax=[]  KbParamMin=[]  KbParamMax=[]  KtParamMin=[]  KtParamMax=[]  POutMin=[]  POutMax=[]  IOutMin=[]  IOutMax=[]  DOutMin=[]  DOutMax=[]  NOutMin=[]  NOutMax=[]  KbOutMin=[]  KbOutMax=[]  KtOutMin=[]  KtOutMax=[]  IntegratorOutMin=[]  IntegratorOutMax=[]  FilterOutMin=[]  FilterOutMax=[]  SumOutMin=[]  SumOutMax=[]  SumI1OutMin=[]  SumI1OutMax=[]  SumI2OutMin=[]  SumI2OutMax=[]  SumI3OutMin=[]  SumI3OutMax=[]  SumDOutMin=[]  SumDOutMax=[]  SaturationOutMin=[]  SaturationOutMax=[]  IntegratorContinuousStateAttributes=''  IntegratorStateMustResolveToSignalObject=off  IntegratorRTWStateStorageClass=Auto  FilterContinuousStateAttributes=''  FilterStateMustResolveToSignalObject=off  FilterRTWStateStorageClass=Auto  DifferentiatorICPrevScaledInput=0  DifferentiatorOutMin=[]  DifferentiatorOutMax=[]  InitialConditionSetting=State (most efficient)
  PID Controller1 : simulink/Continuous/PID Controller  Controller=P  TimeDomain=Continuous-time  SampleTime=-1  IntegratorMethod=Forward Euler  FilterMethod=Forward Euler  Form=Parallel  UseFilter=on  ControllerParametersSource=internal  P=1  I=1  D=0  N=100  InitialConditionSource=internal  InitialConditionForIntegrator=0  InitialConditionForFilter=0  ExternalReset=none  LimitOutput=off  UpperSaturationLimit=inf  LowerSaturationLimit=-inf  LinearizeAsGain=on  AntiWindupMode=none  Kb=1  TrackingMode=off  Kt=1  PParamMin=[]  PParamMax=[]  IParamMin=[]  IParamMax=[]  DParamMin=[]  DParamMax=[]  NParamMin=[]  NParamMax=[]  KbParamMin=[]  KbParamMax=[]  KtParamMin=[]  KtParamMax=[]  POutMin=[]  POutMax=[]  IOutMin=[]  IOutMax=[]  DOutMin=[]  DOutMax=[]  NOutMin=[]  NOutMax=[]  KbOutMin=[]  KbOutMax=[]  KtOutMin=[]  KtOutMax=[]  IntegratorOutMin=[]  IntegratorOutMax=[]  FilterOutMin=[]  FilterOutMax=[]  SumOutMin=[]  SumOutMax=[]  SumI1OutMin=[]  SumI1OutMax=[]  SumI2OutMin=[]  SumI2OutMax=[]  SumI3OutMin=[]  SumI3OutMax=[]  SumDOutMin=[]  SumDOutMax=[]  SaturationOutMin=[]  SaturationOutMax=[]  IntegratorContinuousStateAttributes=''  IntegratorStateMustResolveToSignalObject=off  IntegratorRTWStateStorageClass=Auto  FilterContinuousStateAttributes=''  FilterStateMustResolveToSignalObject=off  FilterRTWStateStorageClass=Auto  DifferentiatorICPrevScaledInput=0  DifferentiatorOutMin=[]  DifferentiatorOutMax=[]  InitialConditionSetting=State (most efficient)
  P_V_comp : Scope  NumInputPorts=6
  Radians to Degrees{1..4} (4 alike) : simulink_extras/Transformations/Radians to Degrees
  Sum : Sum  Inputs=|+-
  Sum1 : Sum  Inputs=++|
  Sum2 : Sum  Inputs=|+-
  Transfer Fcn2 : discretizing/Discretized Transfer Fcn  Commented=on  Numerator=[100]  Denominator=[1 100]  AbsTol=auto  SampleTime=0.001  method=tustin  Wc=1
  TQ : Outport
  wires:
  FFWD/1 -> Sum1/1
  CMD_POS/1 -> [Pcmd], Sum/1
  MEAS_VEL/1 -> [Vmea], Sum2/2  "VEL_meas"
  MEAS_POS/1 -> [Pmea], Sum/2  "POS"
  Sum2/1 -> PID Controller1/1, [Verr]  "Vel_err"
  Manual Switch/1 -> Sum2/1  "Vel_cmd"
  Constant/1 -> Manual Switch/1
  Sum/1 -> PID Controller/1, [Perr]  "Pos_err"
  PID Controller/1 -> Manual Switch/2, [Vcmd]
  Sum1/1 -> TQ/1, [T]
  Mux/1 -> Radians to Degrees4/1
  [Pcmd] -> Mux/1
  [Pmea] -> Mux/2
  Mux1/1 -> Radians to Degrees1/1
  [Vcmd] -> Mux1/1
  [Vmea] -> Mux1/2
  [Verr] -> Radians to Degrees3/1
  [Perr] -> Radians to Degrees2/1
  Radians to Degrees3/1 -> P_V_comp/4  "Vel_err"
  Radians to Degrees2/1 -> P_V_comp/2  "Pos_err"
  Radians to Degrees1/1 -> P_V_comp/3  "Vel"
  Radians to Degrees4/1 -> P_V_comp/1  "Pos"
  [TQ] -> P_V_comp/5  "VTQ"
  [T] -> P_V_comp/6  "T_tot"
  PID Controller1/1 -> Sum1/2, [TQ]
